simulink model "sampleModel1396_4_sub_sub_sub"  (R2023a)
settings: Solver=VariableStepAuto  StartTime=0.0  StopTime=10.0  RelTol=1e-3
libraries: hdlsllib x7, simulink x3
settings Model: Creator=user1  LastModifiedBy=user1

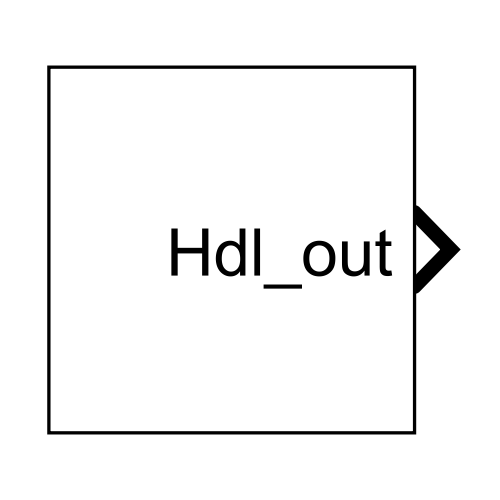
[thumbnail: Simulink's stored preview of the top-level diagram]
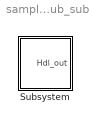
== system sampleModel1396_4_sub_sub_sub ==
  Subsystem : Subsystem

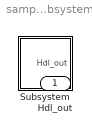
== system sampleModel1396_4_sub_sub_sub/Subsystem ==
  Subsystem : Subsystem
  Hdl_out : Outport  OutDataTypeStr=uint8

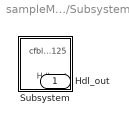
== system sampleModel1396_4_sub_sub_sub/Subsystem/Subsystem ==
  Subsystem : Subsystem
  Hdl_out : Outport  OutDataTypeStr=uint8

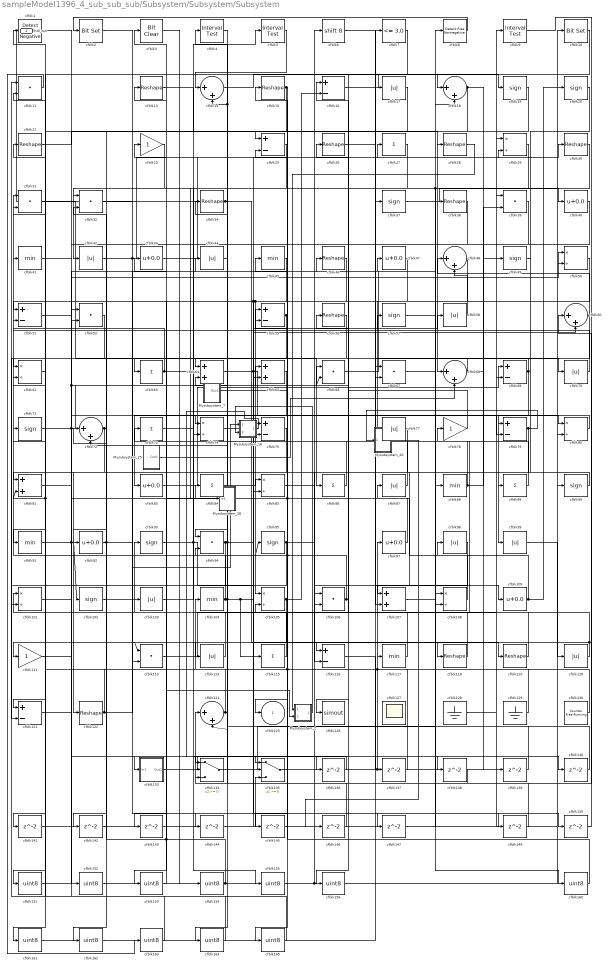
== system sampleModel1396_4_sub_sub_sub/Subsystem/Subsystem/Subsystem ==
  Mysubsystem_16 : Subsystem  TreatAsAtomicUnit=on  RTWFcnName=Mysubsystem_16
      settings: RTWFcnNameOpts=User specified  RTWFileNameOpts=Use function name
  Mysubsystem_2 : Subsystem  TreatAsAtomicUnit=on  RTWFcnName=Mysubsystem_2
      settings: RTWFcnNameOpts=User specified  RTWFileNameOpts=Use function name
  Mysubsystem_20 : Subsystem  TreatAsAtomicUnit=on  RTWFcnName=Mysubsystem_20
      settings: RTWFcnNameOpts=User specified  RTWFileNameOpts=Use function name
  Mysubsystem_25 : Subsystem  TreatAsAtomicUnit=on  RTWFcnName=Mysubsystem_25
      settings: RTWFcnNameOpts=User specified  RTWFileNameOpts=Use function name
  Mysubsystem_28 : Subsystem  TreatAsAtomicUnit=on  RTWFcnName=Mysubsystem_28
      settings: RTWFcnNameOpts=User specified  RTWFileNameOpts=Use function name
  Mysubsystem_7 : Subsystem  TreatAsAtomicUnit=on  RTWFcnName=Mysubsystem_7
      settings: RTWFcnNameOpts=User specified  RTWFileNameOpts=Use function name
  cfblk1 : hdlsllib/Logic and Bit Operations/Detect Fall Negative  vinit=0  OutDataTypeStr=uint8
  cfblk10 : simulink/Logic and Bit Operations/Bit Set  iBit=0
      settings: LibrarySourceBlock=|
      | hdlsllib/Logic and Bit
      | Operations/Bit Set
  cfblk{29,50,61,74,80,85,101,105,108} (9 alike) : Product  Inputs=*/  OutDataTypeStr=uint8  RndMeth=Zero  SaturateOnIntegerOverflow=on
  cfblk{19..20,37,49,57,71,90,93,95,102} (10 alike) : Signum
  cfblk{17,42,44,58,70,77,87,98..99,103,114,120} (12 alike) : Abs  OutDataTypeStr=uint8  SaturateOnIntegerOverflow=off
  cfblk{41,45,88,91,104,117} (6 alike) : MinMax  OutDataTypeStr=uint8
  cfblk{11,31..32,39,52,66..67,94,106,113} (10 alike) : DotProduct  OutDataTypeStr=uint8
  cfblk{64..65,81,107} (4 alike) : Sum  OutDataTypeStr=uint8
  cfblk{40,43,47,83,92,97,109} (7 alike) : Bias  Bias=0.0  SaturateOnIntegerOverflow=off
  cfblk111 : Gain  OutDataTypeStr=uint8
  cfblk{27,63,73,84,86,89,115} (7 alike) : Sum  Inputs=+  OutDataTypeStr=uint8
  cfblk{16,25,51,55,69,75,79,116,121} (9 alike) : Sum  Inputs=+-  OutDataTypeStr=uint8
  cfblk{13,15,21,26,28,30,34,38,46,56,118..119,122} (13 alike) : Reshape
  cfblk{14,18,48,60,68,72,124} (7 alike) : Sum  Inputs=|++  OutDataTypeStr=uint8
  cfblk126 : ToWorkspace  VariableName=simout  SaveFormat=Timeseries  SampleTime=-1
  cfblk127 : Scope
      settings: Floating=on
  cfblk128 : Ground
  cfblk129 : Ground
  cfblk130 : hdlsllib/Sources/Counter Free-Running  NumBits=16  tsamp=-1
  cfblk133 : Subsystem
      settings: LibrarySourceBlock=|
      | hdlsllib/Ports &
      | Subsystems/Subsystem
  cfblk134 : Switch  OutDataTypeStr=uint8  SaturateOnIntegerOverflow=off  InputSameDT=off
  cfblk135 : Switch  OutDataTypeStr=uint8  SaturateOnIntegerOverflow=off  InputSameDT=off
  cfblk{136..147,149..150} (14 alike) : Delay  SampleTime=1
  cfblk{151..156,160..165} (12 alike) : DataTypeConversion  OutDataTypeStr=uint8  SaturateOnIntegerOverflow=off  RndMeth=Floor
  cfblk2 : simulink/Logic and Bit Operations/Bit Set  iBit=0
      settings: LibrarySourceBlock=|
      | hdlsllib/Logic and Bit
      | Operations/Bit Set
  cfblk23 : Gain  OutDataTypeStr=uint8
  cfblk3 : simulink/Logic and Bit Operations/Bit Clear  iBit=0
      settings: LibrarySourceBlock=|
      | hdlsllib/Logic and Bit
      | Operations/Bit Clear
  cfblk4 : hdlsllib/Logic and Bit Operations/Interval Test  IntervalClosedRight=on  uplimit=0.5  IntervalClosedLeft=on  lowlimit=-0.5  OutDataTypeStr=uint8
  cfblk5 : hdlsllib/Logic and Bit Operations/Interval Test  IntervalClosedRight=on  uplimit=0.5  IntervalClosedLeft=on  lowlimit=-0.5  OutDataTypeStr=uint8
  cfblk6 : ArithShift  BitShiftNumber=8
  cfblk7 : hdlsllib/Logic and Bit Operations/Compare To Constant  relop=<=  const=3.0  OutDataTypeStr=uint8
  cfblk78 : Gain  OutDataTypeStr=uint8
  cfblk8 : hdlsllib/Logic and Bit Operations/Detect Rise Nonnegative  vinit=0  OutDataTypeStr=uint8
  cfblk9 : hdlsllib/Logic and Bit Operations/Interval Test  IntervalClosedRight=on  uplimit=0.5  IntervalClosedLeft=on  lowlimit=-0.5  OutDataTypeStr=uint8
  cfblk125 : Outport  OutDataTypeStr=uint8  VectorParamsAs1DForOutWhenUnconnected=off
  Hdl_out : Outport  Port=2  OutDataTypeStr=uint8
  wires:
  cfblk46/1 -> cfblk105/1, cfblk143/1, cfblk85/2
  cfblk8/1 -> cfblk2/1
  cfblk129/1 -> cfblk104/1
  cfblk3/1 -> cfblk154/1
  cfblk16/1 -> cfblk18/1
  cfblk80/1 -> cfblk75/1
  cfblk34/1 -> Hdl_out/1, cfblk118/1
  cfblk70/1 -> cfblk31/1
  cfblk83/1 -> cfblk69/1
  cfblk72/1 -> cfblk142/1, cfblk122/1
  cfblk122/1 -> cfblk51/2, cfblk47/1
  cfblk121/1 -> cfblk46/1
  cfblk31/1 -> cfblk86/1
  cfblk71/1 -> cfblk79/2, cfblk65/1
  cfblk97/1 -> cfblk73/1, cfblk45/1
  cfblk64/1 -> cfblk147/1, cfblk57/1, cfblk99/1
  cfblk113/1 -> cfblk69/2
  cfblk27/1 -> cfblk42/1
  cfblk95/1 -> cfblk113/2, cfblk119/1
  cfblk15/1 -> cfblk145/1, cfblk32/1
  cfblk87/1 -> cfblk15/1
  cfblk67/1 -> cfblk160/1
  cfblk106/1 -> cfblk16/1, cfblk41/1
  cfblk135/1 -> cfblk39/1, cfblk97/1
  cfblk94/1 -> cfblk121/2, cfblk64/2, cfblk27/1
  cfblk37/1 -> cfblk40/1
  cfblk55/1 -> cfblk101/2, cfblk125/1
  cfblk19/1 -> cfblk68/1
  cfblk60/1 -> cfblk91/1, cfblk48/1
  cfblk92/1 -> cfblk72/1, Mysubsystem_16/1(In1)
  cfblk120/1 -> cfblk113/1, cfblk78/1
  cfblk128/1 -> cfblk9/1
  cfblk111/1 -> cfblk84/1
  cfblk65/1 -> cfblk83/1
  cfblk9/1 -> cfblk124/1
  cfblk66/1 -> cfblk30/1
  cfblk89/1 -> cfblk55/1
  cfblk102/1 -> cfblk93/1
  cfblk119/1 -> cfblk66/1
  cfblk90/1 -> cfblk81/1
  cfblk48/1 -> cfblk116/1
  cfblk39/1 -> cfblk126/1
  cfblk61/1 -> cfblk111/1
  cfblk50/1 -> cfblk77/1
  cfblk84/1 -> cfblk85/1
  cfblk130/1 -> cfblk117/1, cfblk101/1, cfblk25/2
  cfblk20/1 -> cfblk89/1
  cfblk109/1 -> cfblk20/1, cfblk87/1
  cfblk85/1 -> cfblk58/1
  cfblk26/1 -> cfblk109/1
  cfblk29/1 -> cfblk108/2, Mysubsystem_28/1(In1)
  cfblk118/1 -> cfblk13/1
  cfblk91/1 -> cfblk50/2, cfblk102/1
  cfblk104/1 -> cfblk31/2, cfblk4/1, cfblk115/1, cfblk60/2
  cfblk47/1 -> cfblk51/1
  cfblk134/1 -> cfblk38/1
  cfblk99/1 -> cfblk120/1
  cfblk78/1 -> cfblk56/1
  cfblk114/1 -> cfblk103/1
  cfblk14/1 -> cfblk19/1
  cfblk117/1 -> cfblk23/1
  cfblk5/1 -> cfblk14/1
  cfblk93/1 -> cfblk150/1, cfblk135/2
  cfblk13/1 -> cfblk28/1
  cfblk6/1 -> cfblk70/1
  cfblk103/1 -> cfblk5/1
  cfblk133/1(Out1) -> cfblk135/1
  cfblk77/1 -> cfblk116/2
  cfblk124/1 -> cfblk34/1, cfblk81/2, cfblk71/1
  cfblk41/1 -> cfblk134/1
  cfblk52/1 -> cfblk61/1
  cfblk69/1 -> cfblk107/2, cfblk63/1
  cfblk105/1 -> cfblk161/1, cfblk16/2
  cfblk40/1 -> cfblk52/2
  cfblk49/1 -> cfblk79/1
  cfblk63/1 -> cfblk138/1, cfblk21/1
  cfblk58/1 -> cfblk48/2
  cfblk44/1 -> cfblk74/1
  cfblk107/1 -> cfblk50/1
  cfblk75/1 -> cfblk94/1
  cfblk68/1 -> cfblk39/2, cfblk64/1
  cfblk74/1 -> cfblk65/2
  cfblk43/1 -> cfblk8/1
  cfblk88/1 -> cfblk49/1, cfblk26/1
  cfblk30/1 -> cfblk74/2
  cfblk101/1 -> cfblk44/1, cfblk66/2
  cfblk115/1 -> cfblk61/2
  cfblk42/1 -> cfblk149/1, cfblk29/2
  cfblk21/1 -> cfblk25/1
  cfblk7/1 -> cfblk151/1
  cfblk18/1 -> cfblk139/1, cfblk92/1
  cfblk1/1 -> cfblk80/1
  cfblk81/1 -> cfblk133/1(In1)
  cfblk57/1 -> cfblk88/1
  cfblk45/1 -> cfblk121/1
  cfblk4/1 -> cfblk14/2, cfblk124/2
  cfblk79/1 -> cfblk107/1, Mysubsystem_20/1(In1)
  cfblk108/1 -> cfblk98/1
  cfblk86/1 -> cfblk43/1
  cfblk38/1 -> cfblk114/1
  cfblk98/1 -> cfblk106/2
  cfblk136/1 -> cfblk134/2
  cfblk116/1 -> cfblk137/1
  cfblk137/1 -> cfblk1/1
  cfblk138/1 -> cfblk134/3
  cfblk139/1 -> cfblk105/2
  cfblk2/1 -> cfblk140/1
  cfblk140/1 -> cfblk72/2
  cfblk17/1 -> cfblk141/1
  cfblk141/1 -> cfblk18/2
  cfblk142/1 -> cfblk135/3
  cfblk143/1 -> cfblk75/2
  cfblk32/1 -> cfblk144/1
  cfblk144/1 -> cfblk29/1
  cfblk145/1 -> cfblk108/1
  cfblk146/1 -> cfblk106/1
  cfblk147/1 -> cfblk80/2
  cfblk149/1 -> cfblk94/2
  cfblk150/1 -> cfblk60/1
  cfblk151/1 -> cfblk6/1, cfblk17/1
  cfblk51/1 -> cfblk152/1
  cfblk152/1 -> cfblk7/1
  cfblk56/1 -> cfblk153/1
  cfblk153/1 -> cfblk3/1
  cfblk154/1 -> cfblk90/1, cfblk32/2, Mysubsystem_2/2(In2)
  cfblk73/1 -> cfblk155/1
  cfblk155/1 -> cfblk10/1
  cfblk10/1 -> cfblk156/1
  cfblk156/1 -> cfblk37/1
  cfblk160/1 -> cfblk95/1, cfblk55/2
  cfblk161/1 -> cfblk67/1
  cfblk23/1 -> cfblk162/1
  cfblk162/1 -> cfblk67/2
  cfblk11/1 -> cfblk163/1
  cfblk163/1 -> cfblk52/1
  cfblk25/1 -> cfblk164/1
  cfblk164/1 -> cfblk11/1
  cfblk165/1 -> cfblk11/2
  cfblk28/1 -> Mysubsystem_2/1(In1)
  Mysubsystem_7/1(Out1) -> cfblk165/1
  Mysubsystem_2/1(Out1) -> Mysubsystem_16/2(In2)
  Mysubsystem_16/1(Out1) -> cfblk136/1
  Mysubsystem_20/1(Out1) -> cfblk146/1
  Mysubsystem_25/1(Out1) -> cfblk68/2

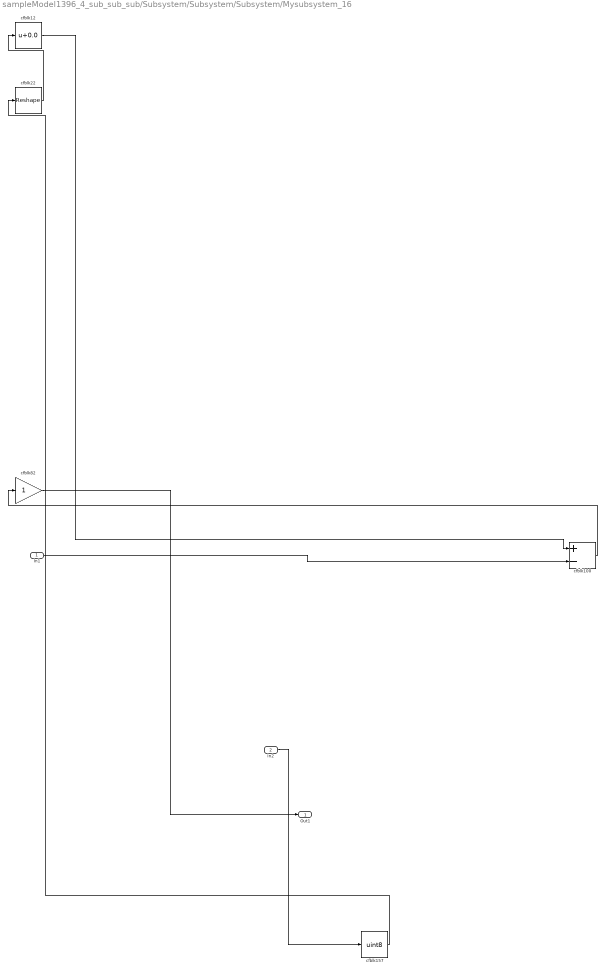
== system sampleModel1396_4_sub_sub_sub/Subsystem/Subsystem/Subsystem/Mysubsystem_16 ==
  In1 : Inport
  In2 : Inport  Port=2
  cfblk100 : Sum  Inputs=+-
  cfblk12 : Bias  Bias=0.0  SaturateOnIntegerOverflow=off
  cfblk157 : DataTypeConversion  OutDataTypeStr=uint8  SaturateOnIntegerOverflow=off  RndMeth=Floor
  cfblk22 : Reshape
  cfblk82 : Gain
  Out1 : Outport
  wires:
  In2/1 -> cfblk157/1
  cfblk157/1 -> cfblk22/1
  In1/1 -> cfblk100/2
  cfblk82/1 -> Out1/1
  cfblk100/1 -> cfblk82/1
  cfblk22/1 -> cfblk12/1
  cfblk12/1 -> cfblk100/1

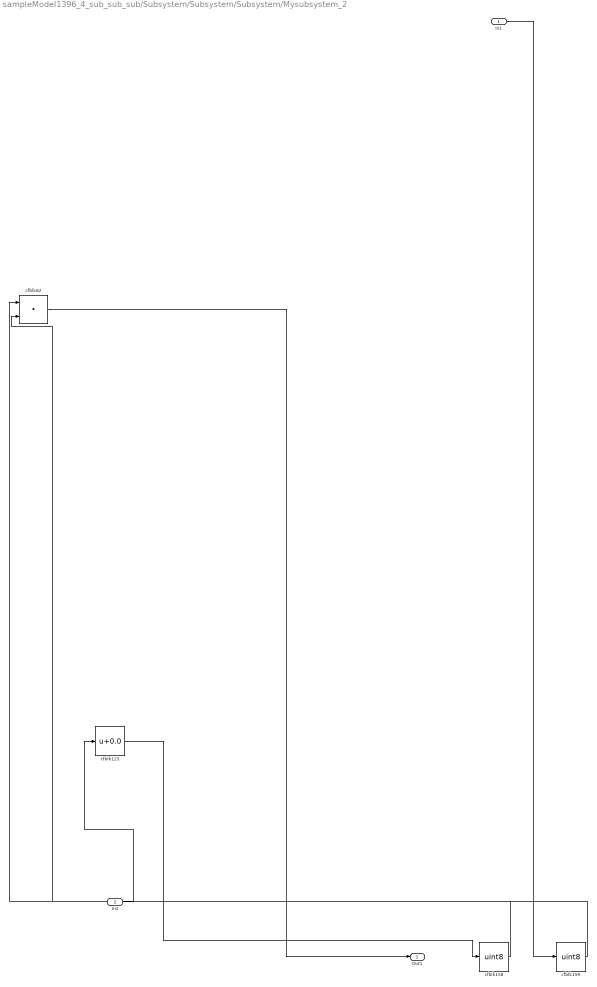
== system sampleModel1396_4_sub_sub_sub/Subsystem/Subsystem/Subsystem/Mysubsystem_2 ==
  In1 : Inport
  In2 : Inport  Port=2
  cfblk123 : Bias  Bias=0.0  SaturateOnIntegerOverflow=off
  cfblk158 : DataTypeConversion  OutDataTypeStr=uint8  SaturateOnIntegerOverflow=off  RndMeth=Floor
  cfblk159 : DataTypeConversion  OutDataTypeStr=uint8  SaturateOnIntegerOverflow=off  RndMeth=Floor
  cfblk62 : DotProduct  OutDataTypeStr=Inherit: Inherit via internal rule
  Out1 : Outport
  wires:
  In1/1 -> cfblk159/1
  In2/1 -> cfblk123/1
  cfblk159/1 -> cfblk62/2
  cfblk158/1 -> cfblk62/1
  cfblk123/1 -> cfblk158/1
  cfblk62/1 -> Out1/1

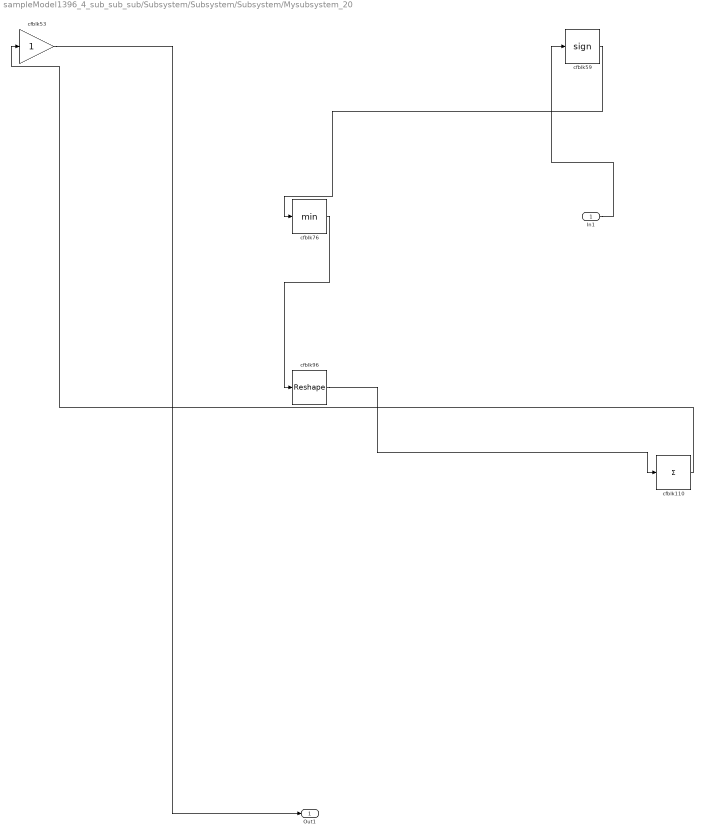
== system sampleModel1396_4_sub_sub_sub/Subsystem/Subsystem/Subsystem/Mysubsystem_20 ==
  In1 : Inport
  cfblk110 : Sum  Inputs=+
  cfblk53 : Gain
  cfblk59 : Signum
  cfblk76 : MinMax
  cfblk96 : Reshape
  Out1 : Outport
  wires:
  In1/1 -> cfblk59/1
  cfblk110/1 -> cfblk53/1
  cfblk53/1 -> Out1/1
  cfblk59/1 -> cfblk76/1
  cfblk96/1 -> cfblk110/1
  cfblk76/1 -> cfblk96/1

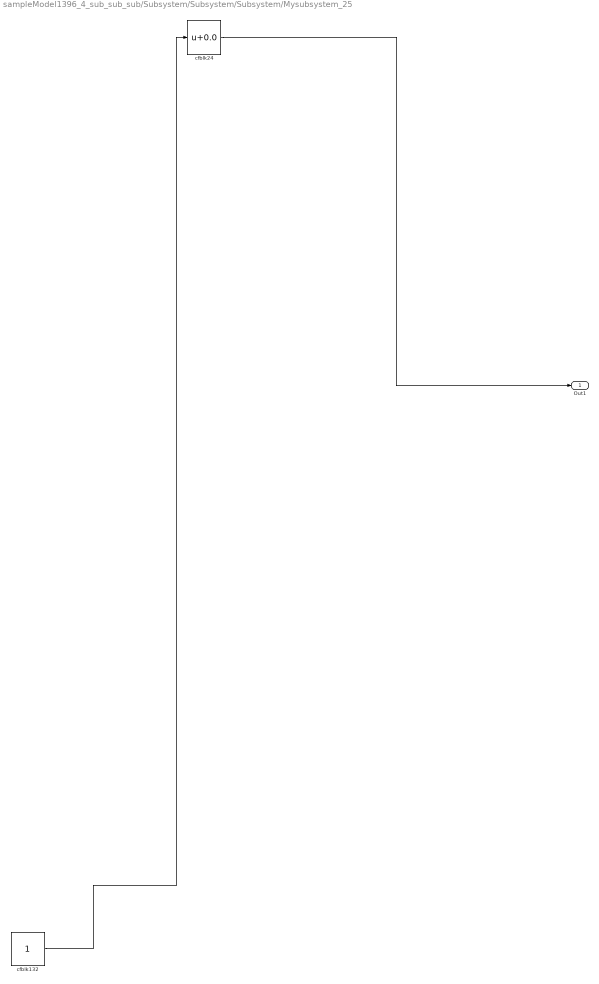
== system sampleModel1396_4_sub_sub_sub/Subsystem/Subsystem/Subsystem/Mysubsystem_25 ==
  cfblk132 : Constant  SampleTime=-1
  cfblk24 : Bias  Bias=0.0  SaturateOnIntegerOverflow=off
  Out1 : Outport
  wires:
  cfblk24/1 -> Out1/1
  cfblk132/1 -> cfblk24/1

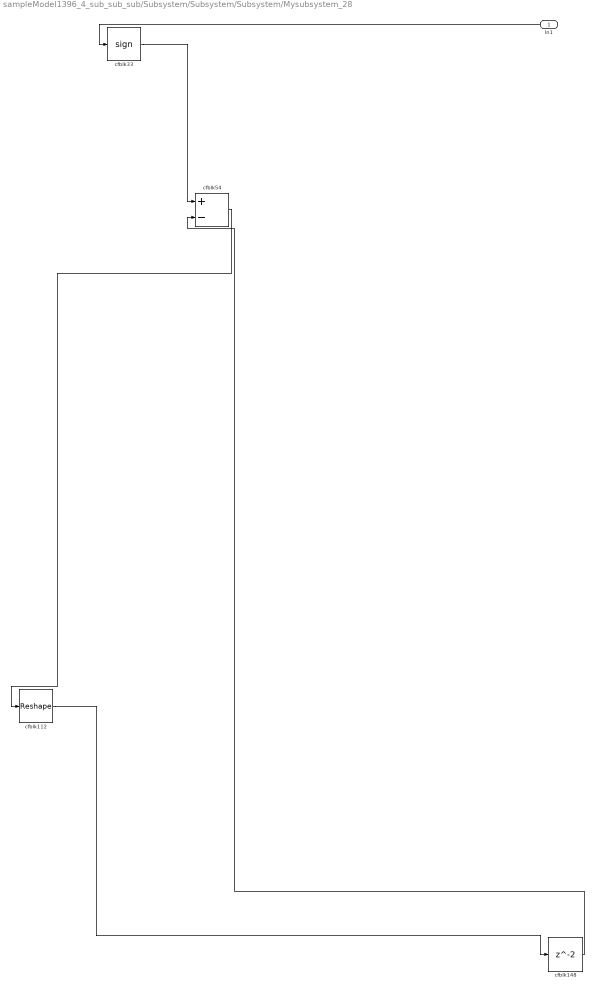
== system sampleModel1396_4_sub_sub_sub/Subsystem/Subsystem/Subsystem/Mysubsystem_28 ==
  In1 : Inport
  cfblk112 : Reshape
  cfblk148 : Delay  SampleTime=1
  cfblk33 : Signum
  cfblk54 : Sum  Inputs=+-
  wires:
  In1/1 -> cfblk33/1
  cfblk33/1 -> cfblk54/1
  cfblk112/1 -> cfblk148/1
  cfblk54/1 -> cfblk112/1
  cfblk148/1 -> cfblk54/2

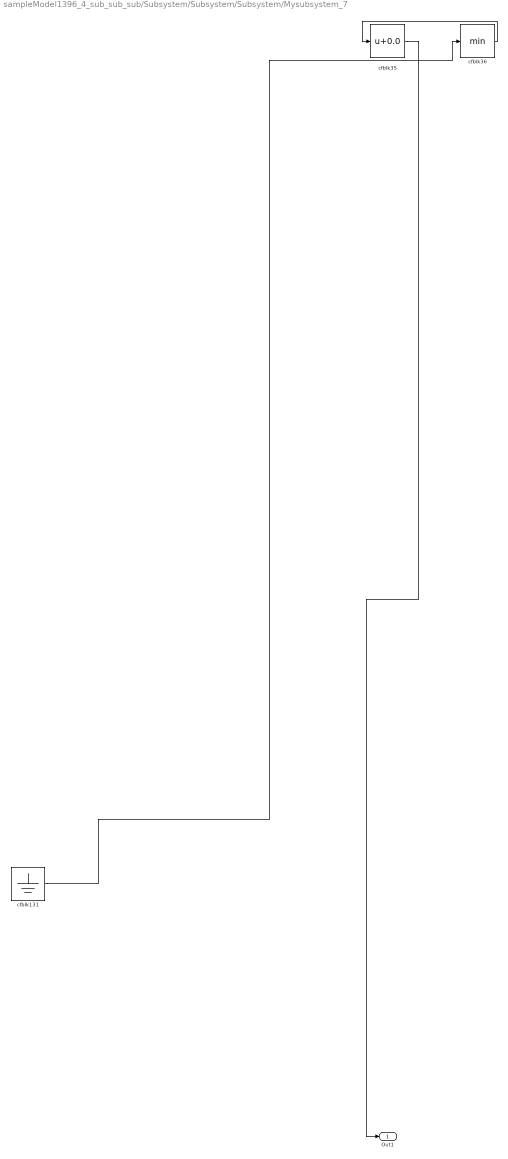
== system sampleModel1396_4_sub_sub_sub/Subsystem/Subsystem/Subsystem/Mysubsystem_7 ==
  cfblk131 : Ground
  cfblk35 : Bias  Bias=0.0  SaturateOnIntegerOverflow=off
  cfblk36 : MinMax
  Out1 : Outport
  wires:
  cfblk35/1 -> Out1/1
  cfblk131/1 -> cfblk36/1
  cfblk36/1 -> cfblk35/1

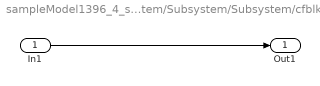
== system sampleModel1396_4_sub_sub_sub/Subsystem/Subsystem/Subsystem/cfblk133 ==
  In1 : Inport
  Out1 : Outport
  wires:
  In1/1 -> Out1/1
